simulink model "Two_area_system_with_wind_farm-DESKTOP-8DA4B7M"  (R2020a)
settings: Solver=ode23tb  StartTime=0.0  StopTime=20  RelTol=1e-3
InitFcn:
  | initAll
values from neighbouring files (symbols this model uses):
  DCgridinit = nDCgrid_init(resultsdc,wB)    [initAll.m]
  Geninit = Generator_init(opdata,SynMach_in_gidx)    [initAll.m]
  SdcgridB = resultsdc.baseMVAdc    [initAll.m]
  SgridB = resultsac.baseMVA    [initAll.m]
  VSCinit = converter_init(resultsac,resultsdc)    [initAll.m]
  wB = 2*pi*fB    (= 314.159265359)    [initAll.m]
undefined symbols (not defined in the file or in its folder): ACgirdinit, AVm0, c1, c2, c3, c4, c5, c6, cp_nom, lambda_nom, P_wind_base, Pelec_base, Pnom, Windinit
libraries: powerlib_meascontrol x9, simulink_extras x1
(part 4 of 4)

== system Two_area_system_with_wind_farm-DESKTOP-8DA4B7M/Generator4/Machine Equations /Interface ==
  delta : Inport
  Vgxy : Inport  Port=2
  Eqd'' : Inport  Port=3
  Bx : Fcn  Expr=1/Xq11+(1/Xd11-1/Xq11)*sin(u(1))*sin(u(1))
  By : Fcn  Expr=-1/Xq11-(1/Xd11-1/Xq11)*cos(u(1))*cos(u(1))
  Gx : Fcn  Expr=(1/Xd11-1/Xq11)*sin(u(1))*cos(u(1))
  Gy : Fcn  Expr=(1/Xq11-1/Xd11)*sin(u(1))*cos(u(1))
  Igx1 : Fcn  Expr=sin(u(1))*u(2)/Xd11-cos(u(1))*u(3)/Xq11
  Igy1 : Fcn  Expr=-cos(u(1))*u(2)/Xd11-sin(u(1))*u(3)/Xq11
  Mux{1..3,5} (4 alike) : Mux  Inputs=2
  Mux4 : Mux
  Scope1 : Scope
  Vdg : Fcn  Expr=u(1)*sin(u(3))-u(2)*cos(u(3))
  Vqg : Fcn  Expr=u(1)*cos(u(3))+u(2)*sin(u(3))
  Vdqg : Outport
  Igxy1 : Outport  Port=2
  GBxy : Outport  Port=3
  wires:
  Vgxy/1 -> Mux1/1
  delta/1 -> By/1, Bx/1, Gy/1, Gx/1, Mux1/2, Mux5/1
  Eqd''/1 -> Mux5/2
  Vdg/1 -> Scope1/1, Mux2/1
  Vqg/1 -> Mux2/2
  Mux2/1 -> Vdqg/1
  Igx1/1 -> Mux3/1
  Igy1/1 -> Mux3/2
  Mux3/1 -> Igxy1/1
  Gx/1 -> Mux4/1
  Gy/1 -> Mux4/2
  Bx/1 -> Mux4/3
  By/1 -> Mux4/4
  Mux4/1 -> GBxy/1
  Mux1/1 -> Vdg/1, Vqg/1
  Mux5/1 -> Igx1/1, Igy1/1

== system Two_area_system_with_wind_farm-DESKTOP-8DA4B7M/Generator4/Machine Equations /Transient Equations ==
  note: Eq
  Idqg : Inport
  Ef : Inport  Port=2
  Trip : Inport  Port=3
  Constant{1..4} (4 alike) : Constant  Value=0
  Ed' : Integrator  InitialCondition=Ed10
  Ed‘’ : Integrator  InitialCondition=Ed110
  Eq' : Integrator  InitialCondition=Eq10
  Eq‘’ : Integrator  InitialCondition=Eq110
  Fcn1 : Fcn  Expr=u(3)-(Xd1-Xd11)*u(1)-u(4)
  Fcn2 : Fcn  Expr=(Xq-Xq1)*u(2)-u(3)
  Fcn3 : Fcn  Expr=-u(1)+(Xq1-Xq11)*u(3)+u(4)
  Fcn7 : Fcn  Expr=u(3)+(Xd-Xd1)*u(1)
  Gain1 : Gain  Gain=1/Td10  SaturateOnIntegerOverflow=on  OutDataTypeStr=Inherit: Same as input  ParamDataTypeStr=Inherit: Same as input
  Gain2 : Gain  Gain=1/Tq0  SaturateOnIntegerOverflow=on  OutDataTypeStr=Inherit: Same as input  ParamDataTypeStr=Inherit: Same as input
  Gain3 : Gain  Gain=1/Td0  SaturateOnIntegerOverflow=on  OutDataTypeStr=Inherit: Same as input  ParamDataTypeStr=Inherit: Same as input
  Gain4 : Gain  Gain=1/Tq10  SaturateOnIntegerOverflow=on  OutDataTypeStr=Inherit: Same as input  ParamDataTypeStr=Inherit: Same as input
  Mux{1..4,6} (5 alike) : Mux  Inputs=2
  Sum1 : Sum  Inputs=|+-  SaturateOnIntegerOverflow=on
  Sum2 : Sum  Inputs=|++  SaturateOnIntegerOverflow=on
  Sum3 : Sum  Inputs=|++  SaturateOnIntegerOverflow=on
  Switch{1..8} (8 alike) : Switch  Criteria=u2 ~= 0  Threshold=0.5  SaturateOnIntegerOverflow=on
  Eqd'' : Outport
  wires:
  Gain3/1 -> Sum2/2, Switch5/3
  Sum1/1 -> Gain3/1
  Mux6/1 -> Fcn7/1, Mux1/1
  Fcn7/1 -> Sum1/2
  Idqg/1 -> Mux2/1, Mux6/1
  Ef/1 -> Sum1/1
  Gain1/1 -> Sum2/1
  Fcn1/1 -> Gain1/1
  Mux1/1 -> Fcn1/1
  Mux2/1 -> Fcn2/1, Mux4/2
  Fcn2/1 -> Gain2/1
  Gain2/1 -> Switch2/3, Sum3/2
  Mux3/1 -> Eqd''/1
  Gain4/1 -> Sum3/1
  Fcn3/1 -> Gain4/1
  Mux4/1 -> Fcn3/1
  Constant1/1 -> Switch2/1, Switch3/1
  Switch2/1 -> Ed'/1
  Ed'/1 -> Switch3/3
  Switch3/1 -> Mux2/2
  Trip/1 -> [Trip]
  [Trip] -> Switch3/2, Switch2/2
  Sum3/1 -> Switch1/3
  Switch1/1 -> Ed‘’/1
  Ed‘’/1 -> Switch4/3
  Switch4/1 -> Mux4/1, Mux3/2
  Constant2/1 -> Switch1/1, Switch4/1
  [Trip] -> Switch4/2, Switch1/2
  Switch5/1 -> Eq'/1
  Eq'/1 -> Switch6/3
  Switch6/1 -> Mux6/2
  Constant3/1 -> Switch6/1, Switch5/1
  [Trip] -> Switch6/2, Switch5/2
  Sum2/1 -> Switch7/3
  Switch7/1 -> Eq‘’/1
  Switch8/1 -> Mux1/2, Mux3/1
  Eq‘’/1 -> Switch8/3
  [Trip] -> Switch8/2, Switch7/2
  Constant4/1 -> Switch7/1, Switch8/1

== system Two_area_system_with_wind_farm-DESKTOP-8DA4B7M/Generator5/Machine Equations /Interface ==
  delta : Inport
  Vgxy : Inport  Port=2
  Eqd'' : Inport  Port=3
  Bx : Fcn  Expr=1/Xq11+(1/Xd11-1/Xq11)*sin(u(1))*sin(u(1))
  By : Fcn  Expr=-1/Xq11-(1/Xd11-1/Xq11)*cos(u(1))*cos(u(1))
  Gx : Fcn  Expr=(1/Xd11-1/Xq11)*sin(u(1))*cos(u(1))
  Gy : Fcn  Expr=(1/Xq11-1/Xd11)*sin(u(1))*cos(u(1))
  Igx1 : Fcn  Expr=sin(u(1))*u(2)/Xd11-cos(u(1))*u(3)/Xq11
  Igy1 : Fcn  Expr=-cos(u(1))*u(2)/Xd11-sin(u(1))*u(3)/Xq11
  Mux{1..3,5} (4 alike) : Mux  Inputs=2
  Mux4 : Mux
  Scope1 : Scope
  Vdg : Fcn  Expr=u(1)*sin(u(3))-u(2)*cos(u(3))
  Vqg : Fcn  Expr=u(1)*cos(u(3))+u(2)*sin(u(3))
  Vdqg : Outport
  Igxy1 : Outport  Port=2
  GBxy : Outport  Port=3
  wires:
  Vgxy/1 -> Mux1/1
  delta/1 -> By/1, Bx/1, Gy/1, Gx/1, Mux1/2, Mux5/1
  Eqd''/1 -> Mux5/2
  Vdg/1 -> Scope1/1, Mux2/1
  Vqg/1 -> Mux2/2
  Mux2/1 -> Vdqg/1
  Igx1/1 -> Mux3/1
  Igy1/1 -> Mux3/2
  Mux3/1 -> Igxy1/1
  Gx/1 -> Mux4/1
  Gy/1 -> Mux4/2
  Bx/1 -> Mux4/3
  By/1 -> Mux4/4
  Mux4/1 -> GBxy/1
  Mux1/1 -> Vdg/1, Vqg/1
  Mux5/1 -> Igx1/1, Igy1/1

== system Two_area_system_with_wind_farm-DESKTOP-8DA4B7M/Generator5/Machine Equations /Transient Equations ==
  note: Eq
  Idqg : Inport
  Ef : Inport  Port=2
  Trip : Inport  Port=3
  Constant{1..4} (4 alike) : Constant  Value=0
  Ed' : Integrator  InitialCondition=Ed10
  Ed‘’ : Integrator  InitialCondition=Ed110
  Eq' : Integrator  InitialCondition=Eq10
  Eq‘’ : Integrator  InitialCondition=Eq110
  Fcn1 : Fcn  Expr=u(3)-(Xd1-Xd11)*u(1)-u(4)
  Fcn2 : Fcn  Expr=(Xq-Xq1)*u(2)-u(3)
  Fcn3 : Fcn  Expr=-u(1)+(Xq1-Xq11)*u(3)+u(4)
  Fcn7 : Fcn  Expr=u(3)+(Xd-Xd1)*u(1)
  Gain1 : Gain  Gain=1/Td10  SaturateOnIntegerOverflow=on  OutDataTypeStr=Inherit: Same as input  ParamDataTypeStr=Inherit: Same as input
  Gain2 : Gain  Gain=1/Tq0  SaturateOnIntegerOverflow=on  OutDataTypeStr=Inherit: Same as input  ParamDataTypeStr=Inherit: Same as input
  Gain3 : Gain  Gain=1/Td0  SaturateOnIntegerOverflow=on  OutDataTypeStr=Inherit: Same as input  ParamDataTypeStr=Inherit: Same as input
  Gain4 : Gain  Gain=1/Tq10  SaturateOnIntegerOverflow=on  OutDataTypeStr=Inherit: Same as input  ParamDataTypeStr=Inherit: Same as input
  Mux{1..4,6} (5 alike) : Mux  Inputs=2
  Sum1 : Sum  Inputs=|+-  SaturateOnIntegerOverflow=on
  Sum2 : Sum  Inputs=|++  SaturateOnIntegerOverflow=on
  Sum3 : Sum  Inputs=|++  SaturateOnIntegerOverflow=on
  Switch{1..8} (8 alike) : Switch  Criteria=u2 ~= 0  Threshold=0.5  SaturateOnIntegerOverflow=on
  Eqd'' : Outport
  wires:
  Gain3/1 -> Sum2/2, Switch5/3
  Sum1/1 -> Gain3/1
  Mux6/1 -> Fcn7/1, Mux1/1
  Fcn7/1 -> Sum1/2
  Idqg/1 -> Mux2/1, Mux6/1
  Ef/1 -> Sum1/1
  Gain1/1 -> Sum2/1
  Fcn1/1 -> Gain1/1
  Mux1/1 -> Fcn1/1
  Mux2/1 -> Fcn2/1, Mux4/2
  Fcn2/1 -> Gain2/1
  Gain2/1 -> Switch2/3, Sum3/2
  Mux3/1 -> Eqd''/1
  Gain4/1 -> Sum3/1
  Fcn3/1 -> Gain4/1
  Mux4/1 -> Fcn3/1
  Constant1/1 -> Switch2/1, Switch3/1
  Switch2/1 -> Ed'/1
  Ed'/1 -> Switch3/3
  Switch3/1 -> Mux2/2
  Trip/1 -> [Trip]
  [Trip] -> Switch3/2, Switch2/2
  Sum3/1 -> Switch1/3
  Switch1/1 -> Ed‘’/1
  Ed‘’/1 -> Switch4/3
  Switch4/1 -> Mux4/1, Mux3/2
  Constant2/1 -> Switch1/1, Switch4/1
  [Trip] -> Switch4/2, Switch1/2
  Switch5/1 -> Eq'/1
  Eq'/1 -> Switch6/3
  Switch6/1 -> Mux6/2
  Constant3/1 -> Switch6/1, Switch5/1
  [Trip] -> Switch6/2, Switch5/2
  Sum2/1 -> Switch7/3
  Switch7/1 -> Eq‘’/1
  Switch8/1 -> Mux1/2, Mux3/1
  Eq‘’/1 -> Switch8/3
  [Trip] -> Switch8/2, Switch7/2
  Constant4/1 -> Switch7/1, Switch8/1

== system Two_area_system_with_wind_farm-DESKTOP-8DA4B7M/VSC1/ control1/control_AC_voltage ==
  usd : Inport
  Enable : EnablePort
  Out_Q_Uac : Subsystem  mask{KP_=Kpac_VSC_A, KI_=Kiac_VSC_A, Upper_limit=inf, Lower_limit=-inf, Upper_saturation_limit=inf, Lower_saturation_limit=-inf, integrator_init=Nq_A_0}
      mask prompts: KP_ "比例系数P"; KI_ "积分系数I"; Upper_limit "限幅上限"; Lower_limit "限幅下限"; Upper_saturation_limit "积分饱和上限"; Lower_saturation_limit "积分饱和下限"; integrator_init "积分初始值"
      mask DialogControl Container4 Prompt: 控制参数
      mask DialogControl Container5 Prompt: 初始值
      mask Display: disp('PI')
  Step : Step  Commented=on  Time=0.5  After=0  SampleTime=0
  Sum13 : Sum  Inputs=|+-  SaturateOnIntegerOverflow=on
  Sum20 : Sum  Inputs=++|  SaturateOnIntegerOverflow=on
  Uref_1 : Constant  Value=Uref
  isqref : Outport
  wires:
  Sum20/1 -> Sum13/1
  Uref_1/1 -> Sum20/2
  Step/1 -> Sum20/1
  Sum13/1 -> Out_Q_Uac/1(In1)
  Out_Q_Uac/1(Out1) -> isqref/1
  usd/1 -> Sum13/2

== system Two_area_system_with_wind_farm-DESKTOP-8DA4B7M/VSC1/ control1/control_P ==
  P : Inport
  Enable : EnablePort
  Out_D_PI : Subsystem  mask{KP_=KpP_VSC_A, KI_=KiP_VSC_A, Upper_limit=inf, Lower_limit=-inf, Upper_saturation_limit=inf, Lower_saturation_limit=-inf, integrator_init=Nd_A_0}
      mask prompts: KP_ "比例系数P"; KI_ "积分系数I"; Upper_limit "限幅上限"; Lower_limit "限幅下限"; Upper_saturation_limit "积分饱和上限"; Lower_saturation_limit "积分饱和下限"; integrator_init "积分初始值"
      mask DialogControl Container4 Prompt: 控制参数
      mask DialogControl Container5 Prompt: 初始值
      mask Display: disp('PI')
  Pref_1 : Constant  Value=Pref
  Scope14 : Scope  NumInputPorts=2
  Step : Step  Commented=on  Time=5  After=-0.5  SampleTime=0
  Sum14 : Sum  Inputs=|+-  SaturateOnIntegerOverflow=on
  Sum19 : Sum  Inputs=++|  SaturateOnIntegerOverflow=on
  isdref : Outport
  wires:
  Pref_1/1 -> Sum19/2
  Sum19/1 -> Sum14/1, Scope14/1
  Sum14/1 -> Out_D_PI/1(In1)
  Out_D_PI/1(Out1) -> isdref/1
  P/1 -> Scope14/2, Sum14/2
  Step/1 -> Sum19/1

== system Two_area_system_with_wind_farm-DESKTOP-8DA4B7M/VSC1/ control1/control_Q ==
  Q : Inport
  Enable : EnablePort
  Out_Q_Q : Subsystem  mask{KP_=KpQ_VSC_A, KI_=KiQ_VSC_A, Upper_limit=inf, Lower_limit=-inf, Upper_saturation_limit=inf, Lower_saturation_limit=-inf, integrator_init=Nq_A_0}
      mask prompts: KP_ "比例系数P"; KI_ "积分系数I"; Upper_limit "限幅上限"; Lower_limit "限幅下限"; Upper_saturation_limit "积分饱和上限"; Lower_saturation_limit "积分饱和下限"; integrator_init "积分初始值"
      mask DialogControl Container4 Prompt: 控制参数
      mask DialogControl Container5 Prompt: 初始值
      mask Display: disp('PI')
  Qref_1 : Constant  Value=Qref
  Scope : Scope  NumInputPorts=2
  Step2 : Step  Commented=on  Time=10  After=0.01  SampleTime=0
  Sum22 : Sum  Inputs=|+-  SaturateOnIntegerOverflow=on
  Sum24 : Sum  Inputs=++|  SaturateOnIntegerOverflow=on
  isqref : Outport
  wires:
  Step2/1 -> Sum24/1
  Sum22/1 -> Out_Q_Q/1(In1)
  Qref_1/1 -> Sum24/2
  Sum24/1 -> Scope/1, Sum22/1
  Out_Q_Q/1(Out1) -> isqref/1
  Q/1 -> Scope/2, Sum22/2

== system Two_area_system_with_wind_farm-DESKTOP-8DA4B7M/VSC1/ control1/control_dc_voltage ==
  udc : Inport
  Enable : EnablePort
  Ground : Ground
  Out_D_Udc : Subsystem  mask{KP_=Kpdc_VSC_A, KI_=Kidc_VSC_A, Upper_limit=inf, Lower_limit=-inf, Upper_saturation_limit=inf, Lower_saturation_limit=-inf, integrator_init=Nd_A_0}
      mask prompts: KP_ "比例系数P"; KI_ "积分系数I"; Upper_limit "限幅上限"; Lower_limit "限幅下限"; Upper_saturation_limit "积分饱和上限"; Lower_saturation_limit "积分饱和下限"; integrator_init "积分初始值"
      mask DialogControl Container4 Prompt: 控制参数
      mask DialogControl Container5 Prompt: 初始值
      mask Display: disp('PI')
  Sum14 : Sum  Inputs=|+-  SaturateOnIntegerOverflow=on
  Sum19 : Sum  Inputs=++|  SaturateOnIntegerOverflow=on
  Udcref_1 : Constant  Value=Udcref
  isdref : Outport
  wires:
  Sum19/1 -> Sum14/1
  udc/1 -> Sum14/2
  Udcref_1/1 -> Sum19/2
  Sum14/1 -> Out_D_Udc/1(In1)
  Ground/1 -> Sum19/1
  Out_D_Udc/1(Out1) -> isdref/1

== system Two_area_system_with_wind_farm-DESKTOP-8DA4B7M/VSC1/ control1/in_D_PI ==
  In1 : Inport
  Ki : Gain  Gain=KI_  SaturateOnIntegerOverflow=on  OutDataTypeStr=Inherit: Same as input  ParamDataTypeStr=Inherit: Same as input
  Kp : Gain  Gain=KP_  SaturateOnIntegerOverflow=on  OutDataTypeStr=Inherit: Same as input  ParamDataTypeStr=Inherit: Same as input
  Saturation2 : Saturate  UpperLimit=Upper_limit  LowerLimit=Lower_limit
  Sum12 : Sum  SaturateOnIntegerOverflow=on
  integrator : Integrator  InitialCondition=integrator_init  LimitOutput=on  UpperSaturationLimit=Upper_saturation_limit  LowerSaturationLimit=Lower_saturation_limit
  Out1 : Outport
  wires:
  In1/1 -> Ki/1, Kp/1
  Kp/1 -> Sum12/2
  Ki/1 -> integrator/1
  integrator/1 -> Sum12/1
  Saturation2/1 -> Out1/1
  Sum12/1 -> Saturation2/1

== system Two_area_system_with_wind_farm-DESKTOP-8DA4B7M/VSC1/ control1/in_Q_PI ==
  In1 : Inport
  Ki : Gain  Gain=KI_  SaturateOnIntegerOverflow=on  OutDataTypeStr=Inherit: Same as input  ParamDataTypeStr=Inherit: Same as input
  Kp : Gain  Gain=KP_  SaturateOnIntegerOverflow=on  OutDataTypeStr=Inherit: Same as input  ParamDataTypeStr=Inherit: Same as input
  Saturation2 : Saturate  UpperLimit=Upper_limit  LowerLimit=Lower_limit
  Sum12 : Sum  SaturateOnIntegerOverflow=on
  integrator : Integrator  InitialCondition=integrator_init  LimitOutput=on  UpperSaturationLimit=Upper_saturation_limit  LowerSaturationLimit=Lower_saturation_limit
  Out1 : Outport
  wires:
  In1/1 -> Ki/1, Kp/1
  Kp/1 -> Sum12/2
  Ki/1 -> integrator/1
  integrator/1 -> Sum12/1
  Saturation2/1 -> Out1/1
  Sum12/1 -> Saturation2/1

== system Two_area_system_with_wind_farm-DESKTOP-8DA4B7M/VSC2/ control1/control_AC_voltage ==
  usd : Inport
  Enable : EnablePort
  Out_Q_Uac : Subsystem  mask{KP_=Kpac_VSC_A, KI_=Kiac_VSC_A, Upper_limit=inf, Lower_limit=-inf, Upper_saturation_limit=inf, Lower_saturation_limit=-inf, integrator_init=Nq_A_0}
      mask prompts: KP_ "比例系数P"; KI_ "积分系数I"; Upper_limit "限幅上限"; Lower_limit "限幅下限"; Upper_saturation_limit "积分饱和上限"; Lower_saturation_limit "积分饱和下限"; integrator_init "积分初始值"
      mask DialogControl Container4 Prompt: 控制参数
      mask DialogControl Container5 Prompt: 初始值
      mask Display: disp('PI')
  Step : Step  Commented=on  Time=0.5  After=0  SampleTime=0
  Sum13 : Sum  Inputs=|+-  SaturateOnIntegerOverflow=on
  Sum20 : Sum  Inputs=++|  SaturateOnIntegerOverflow=on
  Uref_1 : Constant  Value=Uref
  isqref : Outport
  wires:
  Sum20/1 -> Sum13/1
  Uref_1/1 -> Sum20/2
  Step/1 -> Sum20/1
  Sum13/1 -> Out_Q_Uac/1(In1)
  Out_Q_Uac/1(Out1) -> isqref/1
  usd/1 -> Sum13/2

== system Two_area_system_with_wind_farm-DESKTOP-8DA4B7M/VSC2/ control1/control_P ==
  P : Inport
  Enable : EnablePort
  Out_D_PI : Subsystem  mask{KP_=KpP_VSC_A, KI_=KiP_VSC_A, Upper_limit=inf, Lower_limit=-inf, Upper_saturation_limit=inf, Lower_saturation_limit=-inf, integrator_init=Nd_A_0}
      mask prompts: KP_ "比例系数P"; KI_ "积分系数I"; Upper_limit "限幅上限"; Lower_limit "限幅下限"; Upper_saturation_limit "积分饱和上限"; Lower_saturation_limit "积分饱和下限"; integrator_init "积分初始值"
      mask DialogControl Container4 Prompt: 控制参数
      mask DialogControl Container5 Prompt: 初始值
      mask Display: disp('PI')
  Pref_1 : Constant  Value=Pref
  Scope14 : Scope  NumInputPorts=2
  Step : Step  Commented=on  Time=5  After=-0.5  SampleTime=0
  Sum14 : Sum  Inputs=|+-  SaturateOnIntegerOverflow=on
  Sum19 : Sum  Inputs=++|  SaturateOnIntegerOverflow=on
  isdref : Outport
  wires:
  Pref_1/1 -> Sum19/2
  Sum19/1 -> Sum14/1, Scope14/1
  Sum14/1 -> Out_D_PI/1(In1)
  Out_D_PI/1(Out1) -> isdref/1
  P/1 -> Scope14/2, Sum14/2
  Step/1 -> Sum19/1

== system Two_area_system_with_wind_farm-DESKTOP-8DA4B7M/VSC2/ control1/control_Q ==
  Q : Inport
  Enable : EnablePort
  Out_Q_Q : Subsystem  mask{KP_=KpQ_VSC_A, KI_=KiQ_VSC_A, Upper_limit=inf, Lower_limit=-inf, Upper_saturation_limit=inf, Lower_saturation_limit=-inf, integrator_init=Nq_A_0}
      mask prompts: KP_ "比例系数P"; KI_ "积分系数I"; Upper_limit "限幅上限"; Lower_limit "限幅下限"; Upper_saturation_limit "积分饱和上限"; Lower_saturation_limit "积分饱和下限"; integrator_init "积分初始值"
      mask DialogControl Container4 Prompt: 控制参数
      mask DialogControl Container5 Prompt: 初始值
      mask Display: disp('PI')
  Qref_1 : Constant  Value=Qref
  Scope : Scope  NumInputPorts=2
  Step2 : Step  Commented=on  Time=10  After=0.01  SampleTime=0
  Sum22 : Sum  Inputs=|+-  SaturateOnIntegerOverflow=on
  Sum24 : Sum  Inputs=++|  SaturateOnIntegerOverflow=on
  isqref : Outport
  wires:
  Step2/1 -> Sum24/1
  Sum22/1 -> Out_Q_Q/1(In1)
  Qref_1/1 -> Sum24/2
  Sum24/1 -> Scope/1, Sum22/1
  Out_Q_Q/1(Out1) -> isqref/1
  Q/1 -> Scope/2, Sum22/2

== system Two_area_system_with_wind_farm-DESKTOP-8DA4B7M/VSC2/ control1/control_dc_voltage ==
  udc : Inport
  Enable : EnablePort
  Ground : Ground
  Out_D_Udc : Subsystem  mask{KP_=Kpdc_VSC_A, KI_=Kidc_VSC_A, Upper_limit=inf, Lower_limit=-inf, Upper_saturation_limit=inf, Lower_saturation_limit=-inf, integrator_init=Nd_A_0}
      mask prompts: KP_ "比例系数P"; KI_ "积分系数I"; Upper_limit "限幅上限"; Lower_limit "限幅下限"; Upper_saturation_limit "积分饱和上限"; Lower_saturation_limit "积分饱和下限"; integrator_init "积分初始值"
      mask DialogControl Container4 Prompt: 控制参数
      mask DialogControl Container5 Prompt: 初始值
      mask Display: disp('PI')
  Sum14 : Sum  Inputs=|+-  SaturateOnIntegerOverflow=on
  Sum19 : Sum  Inputs=++|  SaturateOnIntegerOverflow=on
  Udcref_1 : Constant  Value=Udcref
  isdref : Outport
  wires:
  Sum19/1 -> Sum14/1
  udc/1 -> Sum14/2
  Udcref_1/1 -> Sum19/2
  Sum14/1 -> Out_D_Udc/1(In1)
  Ground/1 -> Sum19/1
  Out_D_Udc/1(Out1) -> isdref/1

== system Two_area_system_with_wind_farm-DESKTOP-8DA4B7M/VSC2/ control1/in_D_PI ==
  In1 : Inport
  Ki : Gain  Gain=KI_  SaturateOnIntegerOverflow=on  OutDataTypeStr=Inherit: Same as input  ParamDataTypeStr=Inherit: Same as input
  Kp : Gain  Gain=KP_  SaturateOnIntegerOverflow=on  OutDataTypeStr=Inherit: Same as input  ParamDataTypeStr=Inherit: Same as input
  Saturation2 : Saturate  UpperLimit=Upper_limit  LowerLimit=Lower_limit
  Sum12 : Sum  SaturateOnIntegerOverflow=on
  integrator : Integrator  InitialCondition=integrator_init  LimitOutput=on  UpperSaturationLimit=Upper_saturation_limit  LowerSaturationLimit=Lower_saturation_limit
  Out1 : Outport
  wires:
  In1/1 -> Ki/1, Kp/1
  Kp/1 -> Sum12/2
  Ki/1 -> integrator/1
  integrator/1 -> Sum12/1
  Saturation2/1 -> Out1/1
  Sum12/1 -> Saturation2/1

== system Two_area_system_with_wind_farm-DESKTOP-8DA4B7M/VSC2/ control1/in_Q_PI ==
  In1 : Inport
  Ki : Gain  Gain=KI_  SaturateOnIntegerOverflow=on  OutDataTypeStr=Inherit: Same as input  ParamDataTypeStr=Inherit: Same as input
  Kp : Gain  Gain=KP_  SaturateOnIntegerOverflow=on  OutDataTypeStr=Inherit: Same as input  ParamDataTypeStr=Inherit: Same as input
  Saturation2 : Saturate  UpperLimit=Upper_limit  LowerLimit=Lower_limit
  Sum12 : Sum  SaturateOnIntegerOverflow=on
  integrator : Integrator  InitialCondition=integrator_init  LimitOutput=on  UpperSaturationLimit=Upper_saturation_limit  LowerSaturationLimit=Lower_saturation_limit
  Out1 : Outport
  wires:
  In1/1 -> Ki/1, Kp/1
  Kp/1 -> Sum12/2
  Ki/1 -> integrator/1
  integrator/1 -> Sum12/1
  Saturation2/1 -> Out1/1
  Sum12/1 -> Saturation2/1

== system Two_area_system_with_wind_farm-DESKTOP-8DA4B7M/VSC3/ control1/control_AC_voltage ==
  usd : Inport
  Enable : EnablePort
  Out_Q_Uac : Subsystem  mask{KP_=Kpac_VSC_A, KI_=Kiac_VSC_A, Upper_limit=inf, Lower_limit=-inf, Upper_saturation_limit=inf, Lower_saturation_limit=-inf, integrator_init=Nq_A_0}
      mask prompts: KP_ "比例系数P"; KI_ "积分系数I"; Upper_limit "限幅上限"; Lower_limit "限幅下限"; Upper_saturation_limit "积分饱和上限"; Lower_saturation_limit "积分饱和下限"; integrator_init "积分初始值"
      mask DialogControl Container4 Prompt: 控制参数
      mask DialogControl Container5 Prompt: 初始值
      mask Display: disp('PI')
  Step : Step  Commented=on  Time=0.5  After=0  SampleTime=0
  Sum13 : Sum  Inputs=|+-  SaturateOnIntegerOverflow=on
  Sum20 : Sum  Inputs=++|  SaturateOnIntegerOverflow=on
  Uref_1 : Constant  Value=Uref
  isqref : Outport
  wires:
  Sum20/1 -> Sum13/1
  Uref_1/1 -> Sum20/2
  Step/1 -> Sum20/1
  Sum13/1 -> Out_Q_Uac/1(In1)
  Out_Q_Uac/1(Out1) -> isqref/1
  usd/1 -> Sum13/2

== system Two_area_system_with_wind_farm-DESKTOP-8DA4B7M/VSC3/ control1/control_P ==
  P : Inport
  Enable : EnablePort
  Out_D_PI : Subsystem  mask{KP_=KpP_VSC_A, KI_=KiP_VSC_A, Upper_limit=inf, Lower_limit=-inf, Upper_saturation_limit=inf, Lower_saturation_limit=-inf, integrator_init=Nd_A_0}
      mask prompts: KP_ "比例系数P"; KI_ "积分系数I"; Upper_limit "限幅上限"; Lower_limit "限幅下限"; Upper_saturation_limit "积分饱和上限"; Lower_saturation_limit "积分饱和下限"; integrator_init "积分初始值"
      mask DialogControl Container4 Prompt: 控制参数
      mask DialogControl Container5 Prompt: 初始值
      mask Display: disp('PI')
  Pref_1 : Constant  Value=Pref
  Scope14 : Scope  NumInputPorts=2
  Step : Step  Commented=on  Time=5  After=-0.5  SampleTime=0
  Sum14 : Sum  Inputs=|+-  SaturateOnIntegerOverflow=on
  Sum19 : Sum  Inputs=++|  SaturateOnIntegerOverflow=on
  isdref : Outport
  wires:
  Pref_1/1 -> Sum19/2
  Sum19/1 -> Sum14/1, Scope14/1
  Sum14/1 -> Out_D_PI/1(In1)
  Out_D_PI/1(Out1) -> isdref/1
  P/1 -> Scope14/2, Sum14/2
  Step/1 -> Sum19/1

== system Two_area_system_with_wind_farm-DESKTOP-8DA4B7M/VSC3/ control1/control_Q ==
  Q : Inport
  Enable : EnablePort
  Out_Q_Q : Subsystem  mask{KP_=KpQ_VSC_A, KI_=KiQ_VSC_A, Upper_limit=inf, Lower_limit=-inf, Upper_saturation_limit=inf, Lower_saturation_limit=-inf, integrator_init=Nq_A_0}
      mask prompts: KP_ "比例系数P"; KI_ "积分系数I"; Upper_limit "限幅上限"; Lower_limit "限幅下限"; Upper_saturation_limit "积分饱和上限"; Lower_saturation_limit "积分饱和下限"; integrator_init "积分初始值"
      mask DialogControl Container4 Prompt: 控制参数
      mask DialogControl Container5 Prompt: 初始值
      mask Display: disp('PI')
  Qref_1 : Constant  Value=Qref
  Scope : Scope  NumInputPorts=2
  Step2 : Step  Commented=on  Time=10  After=0.01  SampleTime=0
  Sum22 : Sum  Inputs=|+-  SaturateOnIntegerOverflow=on
  Sum24 : Sum  Inputs=++|  SaturateOnIntegerOverflow=on
  isqref : Outport
  wires:
  Step2/1 -> Sum24/1
  Sum22/1 -> Out_Q_Q/1(In1)
  Qref_1/1 -> Sum24/2
  Sum24/1 -> Scope/1, Sum22/1
  Out_Q_Q/1(Out1) -> isqref/1
  Q/1 -> Scope/2, Sum22/2

== system Two_area_system_with_wind_farm-DESKTOP-8DA4B7M/VSC3/ control1/control_dc_voltage ==
  udc : Inport
  Enable : EnablePort
  Ground : Ground
  Out_D_Udc : Subsystem  mask{KP_=Kpdc_VSC_A, KI_=Kidc_VSC_A, Upper_limit=inf, Lower_limit=-inf, Upper_saturation_limit=inf, Lower_saturation_limit=-inf, integrator_init=Nd_A_0}
      mask prompts: KP_ "比例系数P"; KI_ "积分系数I"; Upper_limit "限幅上限"; Lower_limit "限幅下限"; Upper_saturation_limit "积分饱和上限"; Lower_saturation_limit "积分饱和下限"; integrator_init "积分初始值"
      mask DialogControl Container4 Prompt: 控制参数
      mask DialogControl Container5 Prompt: 初始值
      mask Display: disp('PI')
  Sum14 : Sum  Inputs=|+-  SaturateOnIntegerOverflow=on
  Sum19 : Sum  Inputs=++|  SaturateOnIntegerOverflow=on
  Udcref_1 : Constant  Value=Udcref
  isdref : Outport
  wires:
  Sum19/1 -> Sum14/1
  udc/1 -> Sum14/2
  Udcref_1/1 -> Sum19/2
  Sum14/1 -> Out_D_Udc/1(In1)
  Ground/1 -> Sum19/1
  Out_D_Udc/1(Out1) -> isdref/1

== system Two_area_system_with_wind_farm-DESKTOP-8DA4B7M/VSC3/ control1/in_D_PI ==
  In1 : Inport
  Ki : Gain  Gain=KI_  SaturateOnIntegerOverflow=on  OutDataTypeStr=Inherit: Same as input  ParamDataTypeStr=Inherit: Same as input
  Kp : Gain  Gain=KP_  SaturateOnIntegerOverflow=on  OutDataTypeStr=Inherit: Same as input  ParamDataTypeStr=Inherit: Same as input
  Saturation2 : Saturate  UpperLimit=Upper_limit  LowerLimit=Lower_limit
  Sum12 : Sum  SaturateOnIntegerOverflow=on
  integrator : Integrator  InitialCondition=integrator_init  LimitOutput=on  UpperSaturationLimit=Upper_saturation_limit  LowerSaturationLimit=Lower_saturation_limit
  Out1 : Outport
  wires:
  In1/1 -> Ki/1, Kp/1
  Kp/1 -> Sum12/2
  Ki/1 -> integrator/1
  integrator/1 -> Sum12/1
  Saturation2/1 -> Out1/1
  Sum12/1 -> Saturation2/1

== system Two_area_system_with_wind_farm-DESKTOP-8DA4B7M/VSC3/ control1/in_Q_PI ==
  In1 : Inport
  Ki : Gain  Gain=KI_  SaturateOnIntegerOverflow=on  OutDataTypeStr=Inherit: Same as input  ParamDataTypeStr=Inherit: Same as input
  Kp : Gain  Gain=KP_  SaturateOnIntegerOverflow=on  OutDataTypeStr=Inherit: Same as input  ParamDataTypeStr=Inherit: Same as input
  Saturation2 : Saturate  UpperLimit=Upper_limit  LowerLimit=Lower_limit
  Sum12 : Sum  SaturateOnIntegerOverflow=on
  integrator : Integrator  InitialCondition=integrator_init  LimitOutput=on  UpperSaturationLimit=Upper_saturation_limit  LowerSaturationLimit=Lower_saturation_limit
  Out1 : Outport
  wires:
  In1/1 -> Ki/1, Kp/1
  Kp/1 -> Sum12/2
  Ki/1 -> integrator/1
  integrator/1 -> Sum12/1
  Saturation2/1 -> Out1/1
  Sum12/1 -> Saturation2/1

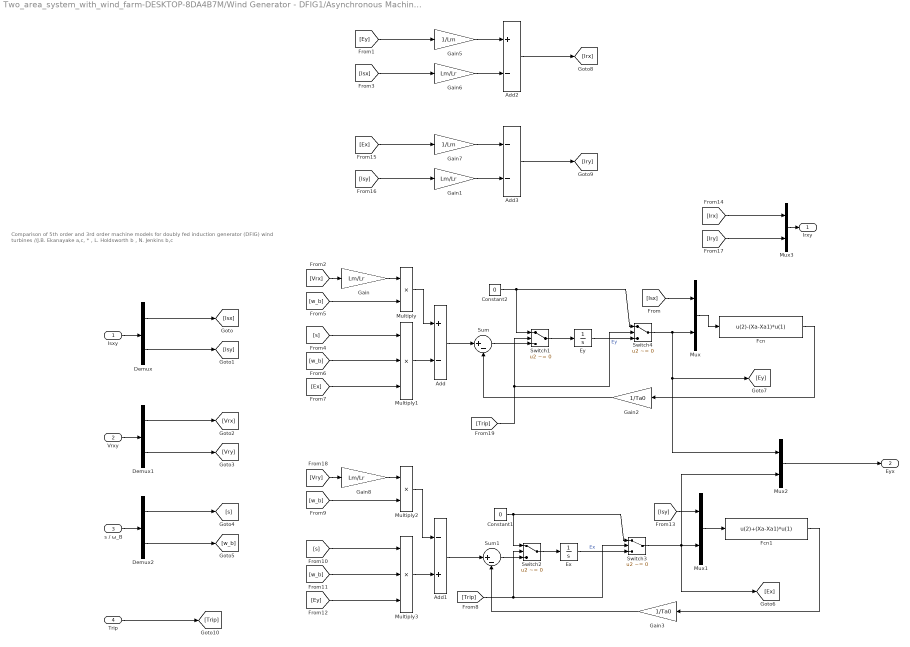
== system Two_area_system_with_wind_farm-DESKTOP-8DA4B7M/Wind Generator - DFIG1/Asynchronous Machine Equations /3th order Transient Equations ==
  note: Comparison of 5th order and 3rd order machine models for doubly fed induction generator (DFIG) wind turbines
      | //J.B. Ekanayake a,c, * , L. Holdsworth b , N. Jenkins b,c
  Isxy : Inport
  Vrxy : Inport  Port=2
  s / ω_B : Inport  Port=3
  Trip : Inport  Port=4
  Add : Sum  Inputs=+-
  Add1 : Sum  Inputs=-+
  Add2 : Sum  Inputs=+-
  Add3 : Sum  Inputs=--
  Constant1 : Constant  Value=0
  Constant2 : Constant  Value=0
  Demux : Demux  Outputs=2
  Demux1 : Demux  Outputs=2
  Demux2 : Demux  Outputs=2
  Ex : Integrator  InitialCondition=Ex0
  Ey : Integrator  InitialCondition=Ey0
  Fcn : Fcn  Expr=u(2)-(Xa-Xa1)*u(1)
  Fcn1 : Fcn  Expr=u(2)+(Xa-Xa1)*u(1)
  Gain{,1,6,8} (4 alike) : Gain  Gain=Lm/Lr
  Gain2 : Gain  Gain=1/Ta0
  Gain3 : Gain  Gain=1/Ta0
  Gain5 : Gain  Gain=1/Lm
  Gain7 : Gain  Gain=1/Lm
  Multiply : Product
  Multiply1 : Product  Inputs=3
  Multiply2 : Product
  Multiply3 : Product  Inputs=3
  Mux{,1..3} (4 alike) : Mux  Inputs=2
  Sum : Sum  Inputs=|+-
  Sum1 : Sum  Inputs=|+-
  Switch{1..4} (4 alike) : Switch  Criteria=u2 ~= 0  Threshold=0.5  SaturateOnIntegerOverflow=on
  Irxy : Outport
  Eyx : Outport  Port=2
  wires:
  [Trip] -> Switch4/2, Switch1/2
  Constant2/1 -> Switch4/1, Switch1/1
  Switch4/1 -> Mux/2, [Ey], Mux2/1
  Ey/1 -> Switch4/3  "Ey"
  Switch1/1 -> Ey/1
  Sum/1 -> Switch1/3
  [Trip] -> Switch2/2, Switch3/2
  Constant1/1 -> Switch3/1, Switch2/1
  Switch3/1 -> Mux1/2, [Ex], Mux2/2
  Ex/1 -> Switch3/3  "Ex"
  Sum1/1 -> Switch2/3
  Switch2/1 -> Ex/1
  Trip/1 -> [Trip]
  [Vry] -> Gain8/1
  Gain8/1 -> Multiply2/1
  Gain/1 -> Multiply/1
  Add3/1 -> [Iry]
  [Isy] -> Gain1/1
  Add2/1 -> [Irx]
  Gain1/1 -> Add3/2
  [Isx] -> Gain6/1
  [Ey] -> Gain5/1
  Gain7/1 -> Add3/1
  [Ex] -> Gain7/1
  Gain6/1 -> Add2/2
  Gain5/1 -> Add2/1
  [Irx] -> Mux3/1
  [Iry] -> Mux3/2
  Mux3/1 -> Irxy/1
  Gain2/1 -> Sum/2
  Gain3/1 -> Sum1/2
  Mux2/1 -> Eyx/1
  Fcn1/1 -> Gain3/1
  Mux1/1 -> Fcn1/1
  [Isy] -> Mux1/1
  Add1/1 -> Sum1/1
  Multiply2/1 -> Add1/1
  Multiply3/1 -> Add1/2
  [s] -> Multiply3/1
  [Ey] -> Multiply3/3
  [w_b] -> Multiply3/2
  [w_b] -> Multiply2/2
  Multiply1/1 -> Add/2
  Add/1 -> Sum/1
  Multiply/1 -> Add/1
  Fcn/1 -> Gain2/1
  Mux/1 -> Fcn/1
  [Isx] -> Mux/1
  [Ex] -> Multiply1/3
  [w_b] -> Multiply1/2
  [s] -> Multiply1/1
  [w_b] -> Multiply/2
  [Vrx] -> Gain/1
  Demux1/2 -> [Vry]
  Demux1/1 -> [Vrx]
  Demux2/2 -> [w_b]
  Demux2/1 -> [s]
  s / ω_B/1 -> Demux2/1
  Vrxy/1 -> Demux1/1
  Isxy/1 -> Demux/1
  Demux/2 -> [Isy]
  Demux/1 -> [Isx]

== system Two_area_system_with_wind_farm-DESKTOP-8DA4B7M/Wind Generator - DFIG1/Asynchronous Machine Equations /Interface ==
  delta : Inport
  Eqd : Inport  Port=2
  Add2 : Sum
  Add3 : Sum
  Bx : Constant  Value=Xa1/( Rs^2+Xa1^2 )
  By : Constant  Value=-Xa1/( Rs^2+Xa1^2 )
  Demux1 : Demux  Outputs=2
  Fcn : Fcn  Expr=(Rs*cos(u(1))+Xa1*sin(u(1))) / (Rs^2+Xa1^2)
  Fcn1 : Fcn  Expr=(Rs*cos(u(1))+Xa1*sin(u(1))) / (Rs^2+Xa1^2)
  Fcn2 : Fcn  Expr=(-Rs*sin(u(1))+Xa1*cos(u(1))) / (Rs^2+Xa1^2)
  Fcn3 : Fcn  Expr=(Rs*sin(u(1))-Xa1*cos(u(1))) / (Rs^2+Xa1^2)
  Gx : Constant  Value=Rs/( Rs^2+Xa1^2 )
  Gy : Constant  Value=Rs/( Rs^2+Xa1^2 )
  Mux3 : Mux  Inputs=2
  Mux4 : Mux
  Product{4..7} (4 alike) : Product
  Igxy1 : Outport
  GBxy : Outport  Port=2
  wires:
  Gx/1 -> Mux4/1
  [gx] -> Product4/1
  [Eq] -> Product5/1
  Product7/1 -> Add3/2
  Product4/1 -> Add2/1
  Product5/1 -> Add2/2
  Add3/1 -> [I1y]
  Product6/1 -> Add3/1
  [Eq] -> Product7/1
  [gy] -> Product7/2
  [bx] -> Product5/2
  Add2/1 -> [I1x]
  [Ed] -> Product6/2
  [Ed] -> Product4/2
  [by] -> Product6/1
  Fcn3/1 -> [by]
  Fcn2/1 -> [bx]
  Fcn1/1 -> [gy]
  Fcn/1 -> [gx]
  [delta] -> Fcn/1, Fcn3/1, Fcn2/1, Fcn1/1
  Demux1/2 -> [Ed]
  Demux1/1 -> [Eq]
  Mux4/1 -> GBxy/1
  By/1 -> Mux4/4
  Bx/1 -> Mux4/3
  Gy/1 -> Mux4/2
  Mux3/1 -> Igxy1/1
  [I1y] -> Mux3/2
  [I1x] -> Mux3/1
  Eqd/1 -> Demux1/1
  delta/1 -> [delta]

== system Two_area_system_with_wind_farm-DESKTOP-8DA4B7M/Wind Generator - DFIG1/Rotor Side Converter control/Power Control ==
  note: $P_s^{ref}=2*(0.5000*\omega_r^2+0.0500*\omega_r+0.1200)$
  wr : Inport
  0-inf1 : Saturate  UpperLimit=inf  LowerLimit=0
  Tracking Curve5 : Fcn  Expr=1.162*u(1)^2
  Ps_ref : Outport
  wires:
  Tracking Curve5/1 -> Ps_ref/1
  0-inf1/1 -> Tracking Curve5/1
  wr/1 -> 0-inf1/1

== system Two_area_system_with_wind_farm-DESKTOP-8DA4B7M/Wind Generator - DFIG1/Rotor Side Converter control/Subsystem ==
  Add5 : Sum  Inputs=++++
  Step : Step  Time=5  After=-0.05  SampleTime=0
  Step1 : Step  Commented=on  Time=22  After=-0.1  SampleTime=0
  Step2 : Step  Commented=on  Time=42  After=-0.1  SampleTime=0
  Step3 : Step  Commented=on  Time=62  After=0.3  SampleTime=0
  Out1 : Outport
  wires:
  Step3/1 -> Add5/4
  Step1/1 -> Add5/2
  Add5/1 -> Out1/1
  Step2/1 -> Add5/3
  Step/1 -> Add5/1

== system Two_area_system_with_wind_farm-DESKTOP-8DA4B7M/Wind Generator - DFIG1/Wind Turbine/Subsystem ==
  wind speed : Inport
  generator speed : Inport  Port=2
  Pitch angle (deg) : Inport  Port=3
  1/cp_nom : Gain  Gain=1/cp_nom  SaturateOnIntegerOverflow=on  OutDataTypeStr=Inherit: Same as input  ParamDataTypeStr=Inherit: Same as input
  Avoid division by zero : Saturate  UpperLimit=1e6  LowerLimit=1e-6
  "Avoid division by zero " : Saturate  UpperLimit=1e6  LowerLimit=1e-6
  Fcn : Fcn  Expr=1/(1/(u[1]+0.08*u[2])-0.035/(u[2]^3+1))
  Fcn1 : Fcn  Expr=c1*(c2/u[2]-c3*u[3]-c4)*exp(-c5/u[2])+c6*u[1]
  Gain : Gain  Gain=-1  SaturateOnIntegerOverflow=on  OutDataTypeStr=Inherit: Same as input  ParamDataTypeStr=Inherit: Same as input
  Mux : Mux  Inputs=2
  Mux1 : Mux  Inputs=3
  Product : Product  Inputs=/*  SaturateOnIntegerOverflow=on  OutDataTypeStr=Inherit: Same as first input
  "Product " : Product  SaturateOnIntegerOverflow=on  OutDataTypeStr=Inherit: Same as first input
  Product1 : Product  Inputs=*/  InputSameDT=on  SaturateOnIntegerOverflow=on  OutDataTypeStr=Inherit: Same as first input
  Saturation1 : Saturate  UpperLimit=inf  LowerLimit=1e-6
  lambda_nom : Gain  Gain=lambda_nom  SaturateOnIntegerOverflow=on  OutDataTypeStr=Inherit: Same as input  ParamDataTypeStr=Inherit: Same as input
  pu->pu : Gain  Gain=P_wind_base*Pnom/Pelec_base  SaturateOnIntegerOverflow=on  OutDataTypeStr=Inherit: Same as input  ParamDataTypeStr=Inherit: Same as input
  wind_speed^3 : Fcn  Expr=u(1)^3
  Tm : Outport
  wires:
  Pitch angle (deg)/1 -> Mux/2, Mux1/3
  Saturation1/1 -> Mux/1, Mux1/1
  Fcn1/1 -> 1/cp_nom/1
  Mux1/1 -> Fcn1/1
  Mux/1 -> Fcn/1
  Fcn/1 -> Mux1/2  "lambda_i"
  Gain/1 -> Tm/1
  Product1/1 -> Gain/1
  "Product "/1 -> pu->pu/1  "Pm_pu"
  lambda_nom/1 -> Saturation1/1
  generator speed/1 -> Avoid division by zero/1, Product/2
  "Avoid division by zero "/1 -> Product/1
  pu->pu/1 -> Product1/1
  Product/1 -> lambda_nom/1
  Avoid division by zero/1 -> Product1/2
  wind_speed^3/1 -> "Product "/1  "Pwind_pu"
  1/cp_nom/1 -> "Product "/2  "cp_pu"
  wind speed/1 -> "Avoid division by zero "/1, wind_speed^3/1  "wind_speed_pu"

== system Two_area_system_with_wind_farm-DESKTOP-8DA4B7M/VSC1/ control1/control_AC_voltage/Out_Q_Uac ==
  In1 : Inport
  Ki : Gain  Gain=KI_  SaturateOnIntegerOverflow=on  OutDataTypeStr=Inherit: Same as input  ParamDataTypeStr=Inherit: Same as input
  Kp : Gain  Gain=KP_  SaturateOnIntegerOverflow=on  OutDataTypeStr=Inherit: Same as input  ParamDataTypeStr=Inherit: Same as input
  Saturation2 : Saturate  UpperLimit=Upper_limit  LowerLimit=Lower_limit
  Sum12 : Sum  SaturateOnIntegerOverflow=on
  integrator : Integrator  InitialCondition=integrator_init  LimitOutput=on  UpperSaturationLimit=Upper_saturation_limit  LowerSaturationLimit=Lower_saturation_limit
  Out1 : Outport
  wires:
  In1/1 -> Ki/1, Kp/1
  Kp/1 -> Sum12/2
  Ki/1 -> integrator/1
  integrator/1 -> Sum12/1
  Saturation2/1 -> Out1/1
  Sum12/1 -> Saturation2/1

== system Two_area_system_with_wind_farm-DESKTOP-8DA4B7M/VSC1/ control1/control_P/Out_D_PI ==
  In1 : Inport
  Ki : Gain  Gain=KI_  SaturateOnIntegerOverflow=on  OutDataTypeStr=Inherit: Same as input  ParamDataTypeStr=Inherit: Same as input
  Kp : Gain  Gain=KP_  SaturateOnIntegerOverflow=on  OutDataTypeStr=Inherit: Same as input  ParamDataTypeStr=Inherit: Same as input
  Saturation2 : Saturate  UpperLimit=Upper_limit  LowerLimit=Lower_limit
  Sum12 : Sum  SaturateOnIntegerOverflow=on
  integrator : Integrator  InitialCondition=integrator_init  LimitOutput=on  UpperSaturationLimit=Upper_saturation_limit  LowerSaturationLimit=Lower_saturation_limit
  Out1 : Outport
  wires:
  In1/1 -> Ki/1, Kp/1
  Ki/1 -> integrator/1
  Kp/1 -> Sum12/2
  integrator/1 -> Sum12/1
  Sum12/1 -> Saturation2/1
  Saturation2/1 -> Out1/1

== system Two_area_system_with_wind_farm-DESKTOP-8DA4B7M/VSC1/ control1/control_Q/Out_Q_Q ==
  In1 : Inport
  Ki : Gain  Gain=KI_  SaturateOnIntegerOverflow=on  OutDataTypeStr=Inherit: Same as input  ParamDataTypeStr=Inherit: Same as input
  Kp : Gain  Gain=KP_  SaturateOnIntegerOverflow=on  OutDataTypeStr=Inherit: Same as input  ParamDataTypeStr=Inherit: Same as input
  Saturation2 : Saturate  UpperLimit=Upper_limit  LowerLimit=Lower_limit
  Sum12 : Sum  SaturateOnIntegerOverflow=on
  integrator : Integrator  InitialCondition=integrator_init  LimitOutput=on  UpperSaturationLimit=Upper_saturation_limit  LowerSaturationLimit=Lower_saturation_limit
  Out1 : Outport
  wires:
  In1/1 -> Ki/1, Kp/1
  Kp/1 -> Sum12/2
  Ki/1 -> integrator/1
  integrator/1 -> Sum12/1
  Saturation2/1 -> Out1/1
  Sum12/1 -> Saturation2/1

== system Two_area_system_with_wind_farm-DESKTOP-8DA4B7M/VSC1/ control1/control_dc_voltage/Out_D_Udc ==
  In1 : Inport
  Ki : Gain  Gain=KI_  SaturateOnIntegerOverflow=on  OutDataTypeStr=Inherit: Same as input  ParamDataTypeStr=Inherit: Same as input
  Kp : Gain  Gain=KP_  SaturateOnIntegerOverflow=on  OutDataTypeStr=Inherit: Same as input  ParamDataTypeStr=Inherit: Same as input
  Saturation2 : Saturate  UpperLimit=Upper_limit  LowerLimit=Lower_limit
  Sum12 : Sum  SaturateOnIntegerOverflow=on
  integrator : Integrator  InitialCondition=integrator_init  LimitOutput=on  UpperSaturationLimit=Upper_saturation_limit  LowerSaturationLimit=Lower_saturation_limit
  Out1 : Outport
  wires:
  In1/1 -> Ki/1, Kp/1
  Ki/1 -> integrator/1
  Kp/1 -> Sum12/2
  integrator/1 -> Sum12/1
  Sum12/1 -> Saturation2/1
  Saturation2/1 -> Out1/1

== system Two_area_system_with_wind_farm-DESKTOP-8DA4B7M/VSC2/ control1/control_AC_voltage/Out_Q_Uac ==
  In1 : Inport
  Ki : Gain  Gain=KI_  SaturateOnIntegerOverflow=on  OutDataTypeStr=Inherit: Same as input  ParamDataTypeStr=Inherit: Same as input
  Kp : Gain  Gain=KP_  SaturateOnIntegerOverflow=on  OutDataTypeStr=Inherit: Same as input  ParamDataTypeStr=Inherit: Same as input
  Saturation2 : Saturate  UpperLimit=Upper_limit  LowerLimit=Lower_limit
  Sum12 : Sum  SaturateOnIntegerOverflow=on
  integrator : Integrator  InitialCondition=integrator_init  LimitOutput=on  UpperSaturationLimit=Upper_saturation_limit  LowerSaturationLimit=Lower_saturation_limit
  Out1 : Outport
  wires:
  In1/1 -> Ki/1, Kp/1
  Kp/1 -> Sum12/2
  Ki/1 -> integrator/1
  integrator/1 -> Sum12/1
  Saturation2/1 -> Out1/1
  Sum12/1 -> Saturation2/1

== system Two_area_system_with_wind_farm-DESKTOP-8DA4B7M/VSC2/ control1/control_P/Out_D_PI ==
  In1 : Inport
  Ki : Gain  Gain=KI_  SaturateOnIntegerOverflow=on  OutDataTypeStr=Inherit: Same as input  ParamDataTypeStr=Inherit: Same as input
  Kp : Gain  Gain=KP_  SaturateOnIntegerOverflow=on  OutDataTypeStr=Inherit: Same as input  ParamDataTypeStr=Inherit: Same as input
  Saturation2 : Saturate  UpperLimit=Upper_limit  LowerLimit=Lower_limit
  Sum12 : Sum  SaturateOnIntegerOverflow=on
  integrator : Integrator  InitialCondition=integrator_init  LimitOutput=on  UpperSaturationLimit=Upper_saturation_limit  LowerSaturationLimit=Lower_saturation_limit
  Out1 : Outport
  wires:
  In1/1 -> Ki/1, Kp/1
  Ki/1 -> integrator/1
  Kp/1 -> Sum12/2
  integrator/1 -> Sum12/1
  Sum12/1 -> Saturation2/1
  Saturation2/1 -> Out1/1

== system Two_area_system_with_wind_farm-DESKTOP-8DA4B7M/VSC2/ control1/control_Q/Out_Q_Q ==
  In1 : Inport
  Ki : Gain  Gain=KI_  SaturateOnIntegerOverflow=on  OutDataTypeStr=Inherit: Same as input  ParamDataTypeStr=Inherit: Same as input
  Kp : Gain  Gain=KP_  SaturateOnIntegerOverflow=on  OutDataTypeStr=Inherit: Same as input  ParamDataTypeStr=Inherit: Same as input
  Saturation2 : Saturate  UpperLimit=Upper_limit  LowerLimit=Lower_limit
  Sum12 : Sum  SaturateOnIntegerOverflow=on
  integrator : Integrator  InitialCondition=integrator_init  LimitOutput=on  UpperSaturationLimit=Upper_saturation_limit  LowerSaturationLimit=Lower_saturation_limit
  Out1 : Outport
  wires:
  In1/1 -> Ki/1, Kp/1
  Kp/1 -> Sum12/2
  Ki/1 -> integrator/1
  integrator/1 -> Sum12/1
  Saturation2/1 -> Out1/1
  Sum12/1 -> Saturation2/1

== system Two_area_system_with_wind_farm-DESKTOP-8DA4B7M/VSC2/ control1/control_dc_voltage/Out_D_Udc ==
  In1 : Inport
  Ki : Gain  Gain=KI_  SaturateOnIntegerOverflow=on  OutDataTypeStr=Inherit: Same as input  ParamDataTypeStr=Inherit: Same as input
  Kp : Gain  Gain=KP_  SaturateOnIntegerOverflow=on  OutDataTypeStr=Inherit: Same as input  ParamDataTypeStr=Inherit: Same as input
  Saturation2 : Saturate  UpperLimit=Upper_limit  LowerLimit=Lower_limit
  Sum12 : Sum  SaturateOnIntegerOverflow=on
  integrator : Integrator  InitialCondition=integrator_init  LimitOutput=on  UpperSaturationLimit=Upper_saturation_limit  LowerSaturationLimit=Lower_saturation_limit
  Out1 : Outport
  wires:
  In1/1 -> Ki/1, Kp/1
  Ki/1 -> integrator/1
  Kp/1 -> Sum12/2
  integrator/1 -> Sum12/1
  Sum12/1 -> Saturation2/1
  Saturation2/1 -> Out1/1

== system Two_area_system_with_wind_farm-DESKTOP-8DA4B7M/VSC3/ control1/control_AC_voltage/Out_Q_Uac ==
  In1 : Inport
  Ki : Gain  Gain=KI_  SaturateOnIntegerOverflow=on  OutDataTypeStr=Inherit: Same as input  ParamDataTypeStr=Inherit: Same as input
  Kp : Gain  Gain=KP_  SaturateOnIntegerOverflow=on  OutDataTypeStr=Inherit: Same as input  ParamDataTypeStr=Inherit: Same as input
  Saturation2 : Saturate  UpperLimit=Upper_limit  LowerLimit=Lower_limit
  Sum12 : Sum  SaturateOnIntegerOverflow=on
  integrator : Integrator  InitialCondition=integrator_init  LimitOutput=on  UpperSaturationLimit=Upper_saturation_limit  LowerSaturationLimit=Lower_saturation_limit
  Out1 : Outport
  wires:
  In1/1 -> Ki/1, Kp/1
  Kp/1 -> Sum12/2
  Ki/1 -> integrator/1
  integrator/1 -> Sum12/1
  Saturation2/1 -> Out1/1
  Sum12/1 -> Saturation2/1

== system Two_area_system_with_wind_farm-DESKTOP-8DA4B7M/VSC3/ control1/control_P/Out_D_PI ==
  In1 : Inport
  Ki : Gain  Gain=KI_  SaturateOnIntegerOverflow=on  OutDataTypeStr=Inherit: Same as input  ParamDataTypeStr=Inherit: Same as input
  Kp : Gain  Gain=KP_  SaturateOnIntegerOverflow=on  OutDataTypeStr=Inherit: Same as input  ParamDataTypeStr=Inherit: Same as input
  Saturation2 : Saturate  UpperLimit=Upper_limit  LowerLimit=Lower_limit
  Sum12 : Sum  SaturateOnIntegerOverflow=on
  integrator : Integrator  InitialCondition=integrator_init  LimitOutput=on  UpperSaturationLimit=Upper_saturation_limit  LowerSaturationLimit=Lower_saturation_limit
  Out1 : Outport
  wires:
  In1/1 -> Ki/1, Kp/1
  Ki/1 -> integrator/1
  Kp/1 -> Sum12/2
  integrator/1 -> Sum12/1
  Sum12/1 -> Saturation2/1
  Saturation2/1 -> Out1/1

== system Two_area_system_with_wind_farm-DESKTOP-8DA4B7M/VSC3/ control1/control_Q/Out_Q_Q ==
  In1 : Inport
  Ki : Gain  Gain=KI_  SaturateOnIntegerOverflow=on  OutDataTypeStr=Inherit: Same as input  ParamDataTypeStr=Inherit: Same as input
  Kp : Gain  Gain=KP_  SaturateOnIntegerOverflow=on  OutDataTypeStr=Inherit: Same as input  ParamDataTypeStr=Inherit: Same as input
  Saturation2 : Saturate  UpperLimit=Upper_limit  LowerLimit=Lower_limit
  Sum12 : Sum  SaturateOnIntegerOverflow=on
  integrator : Integrator  InitialCondition=integrator_init  LimitOutput=on  UpperSaturationLimit=Upper_saturation_limit  LowerSaturationLimit=Lower_saturation_limit
  Out1 : Outport
  wires:
  In1/1 -> Ki/1, Kp/1
  Kp/1 -> Sum12/2
  Ki/1 -> integrator/1
  integrator/1 -> Sum12/1
  Saturation2/1 -> Out1/1
  Sum12/1 -> Saturation2/1

== system Two_area_system_with_wind_farm-DESKTOP-8DA4B7M/VSC3/ control1/control_dc_voltage/Out_D_Udc ==
  In1 : Inport
  Ki : Gain  Gain=KI_  SaturateOnIntegerOverflow=on  OutDataTypeStr=Inherit: Same as input  ParamDataTypeStr=Inherit: Same as input
  Kp : Gain  Gain=KP_  SaturateOnIntegerOverflow=on  OutDataTypeStr=Inherit: Same as input  ParamDataTypeStr=Inherit: Same as input
  Saturation2 : Saturate  UpperLimit=Upper_limit  LowerLimit=Lower_limit
  Sum12 : Sum  SaturateOnIntegerOverflow=on
  integrator : Integrator  InitialCondition=integrator_init  LimitOutput=on  UpperSaturationLimit=Upper_saturation_limit  LowerSaturationLimit=Lower_saturation_limit
  Out1 : Outport
  wires:
  In1/1 -> Ki/1, Kp/1
  Ki/1 -> integrator/1
  Kp/1 -> Sum12/2
  integrator/1 -> Sum12/1
  Sum12/1 -> Saturation2/1
  Saturation2/1 -> Out1/1
